simulink subsystem "Modelo_Motores"  (R2023b)
settings: Solver=VariableStepAuto  StartTime=0.0  StopTime=10.0  RelTol=1e-3
libraries: arduinolib x6, simulink x2
settings Model: Creator=Claudia Ada  LastModifiedBy=pablo

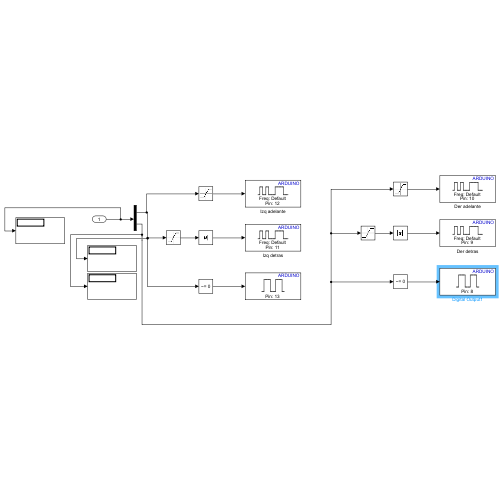
[thumbnail: Simulink's stored preview of the top-level diagram]
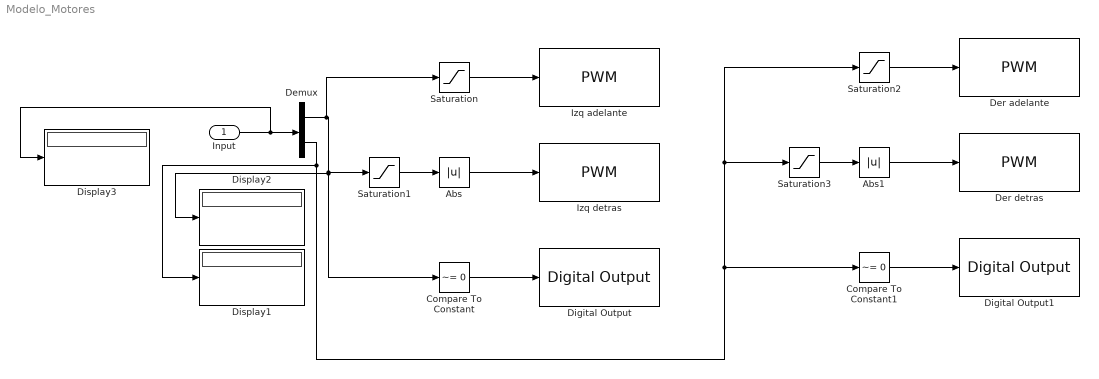
== system Modelo_Motores ==
  Input : Inport
  Abs : Abs  SaturateOnIntegerOverflow=off
  Abs1 : Abs  SaturateOnIntegerOverflow=off
  Compare To Constant : simulink/Logic and Bit Operations/Compare To Constant  relop=~=  const=0  OutDataTypeStr=boolean
  Compare To Constant1 : simulink/Logic and Bit Operations/Compare To Constant  relop=~=  const=0  OutDataTypeStr=boolean
  Demux : Demux  Outputs=2
  Der adelante : arduinolib/PWM  pinNumber=10  frequencyType=Default  desiredFrequency=490.2  achievableFrequency=490.2
  Der detras : arduinolib/PWM  pinNumber=9  frequencyType=Default  desiredFrequency=490.2  achievableFrequency=490.2
  Digital Output : arduinolib/Digital Output  pinNumber=13  Direction=output  blockPlatform=arduino
  Digital Output1 : arduinolib/Digital Output  pinNumber=8  Direction=output  blockPlatform=arduino
  Display1 : Display
  Display2 : Display
  Display3 : Display
  Izq adelante : arduinolib/PWM  pinNumber=12  frequencyType=Default  desiredFrequency=490.2  achievableFrequency=490.2
  Izq detras : arduinolib/PWM  pinNumber=11  frequencyType=Default  desiredFrequency=490.2  achievableFrequency=490.2
  Saturation : Saturate  UpperLimit=100  LowerLimit=0
  Saturation1 : Saturate  UpperLimit=0  LowerLimit=-100
  Saturation2 : Saturate  UpperLimit=100  LowerLimit=0
  Saturation3 : Saturate  UpperLimit=0  LowerLimit=-100
  wires:
  Saturation/1 -> Izq adelante/1
  Saturation1/1 -> Abs/1
  Abs/1 -> Izq detras/1
  Compare To Constant/1 -> Digital Output/1
  Input/1 -> Demux/1, Display3/1
  Saturation2/1 -> Der adelante/1
  Abs1/1 -> Der detras/1
  Saturation3/1 -> Abs1/1
  Compare To Constant1/1 -> Digital Output1/1
  Demux/1 -> Saturation1/1, Display2/1, Compare To Constant/1, Saturation/1
  Demux/2 -> Saturation2/1, Saturation3/1, Compare To Constant1/1, Display1/1
